simulink model "pendulum_model_2200mAh"  (R2017a)
settings: Solver=FixedStepAuto  StartTime=0.0  StopTime=12  FixedStep=0.01  RelTol=1e-3
values from neighbouring files (symbols this model uses):
  c = params(1)    [Swing_Test_Graph_2200mAh.m]
  g = 9.81    [Swing_Test_Graph_2200mAh.m]    (also in leastSquares.m)
  I = params(2)    [Swing_Test_Graph_2200mAh.m]
  l = 0.111    [Swing_Test_Graph_2200mAh.m]    (also in leastSquares.m)
  M = 0.437    [Swing_Test_Graph_2200mAh.m]    (also in leastSquares.m)
  theta0 = 1.09    [Swing_Test_Graph_2200mAh.m]
settings Model: Creator=Patrick  LastModifiedBy=Patrick
settings DataIOCC: TimeSaveName=tsim

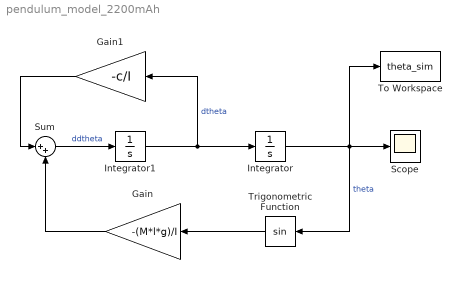
== system pendulum_model_2200mAh ==
  Gain : Gain  Gain=-(M*l*g)/I
  Gain1 : Gain  Gain=-c/I
  Integrator : Integrator  InitialCondition=theta0
  Integrator1 : Integrator
  Scope : Scope
  Sum : Sum  Inputs=|++
  To Workspace : ToWorkspace  VariableName=theta_sim  SampleTime=-1
  Trigonometric Function : Trigonometry
  wires:
  Integrator/1 -> To Workspace/1, Scope/1, Trigonometric Function/1  "theta"
  Integrator1/1 -> Integrator/1, Gain1/1  "dtheta"
  Trigonometric Function/1 -> Gain/1
  Sum/1 -> Integrator1/1  "ddtheta"
  Gain1/1 -> Sum/1
  Gain/1 -> Sum/2
